simulink library "dspsigattribs"  (Simulink 8.0)
settings: Solver=ode45  SolverMode=SingleTasking  StartTime=0.0  StopTime=10.0  RelTol=1e-3
values from neighbouring files (symbols this model uses):
  D = D + B    [rebuffer_delay.m]
libraries: simulink x2
settings Model: RequirementInfo=9  Creator=don  LastModifiedBy=lij  CovMetricSettings=d  ExtModeAutoUpdateStatusClock=off
settings Model: ForwardingTableString=|
  | ||__slOldName__||dspsigattribs/Contiguous
  | Copy||__slNewName__||dspobslib/Contiguous
  | Copy||__slOldName__||dspsigattribs/Frame Status
  | Conversion||__slNewName__||dspobslib/Frame Status
  | Conversion

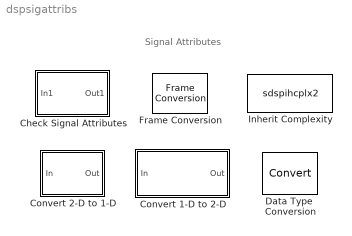
== system dspsigattribs ==
  note: Signal Attributes
  Check Signal Attributes : Subsystem  mask(Check Signal Attributes){SigAttribCheckMethod=Does not match attributes exactly, Complexity=Ignore, Frame=Ignore, DimsCheckMethod=Ignore, Dimensions=1-D, DatatypeCheckMethod=Ignore, DatatypeGeneral=Boolean, DtypeFloatSpecific=Any floating-point, DtypeFixedSpecific=Any fixed-point, DtypeIntSpecific=Any integer, SampleMode=Ignore}
      mask prompts: SigAttribCheckMethod "Error when input:"; Frame "Frame status:"; DimsCheckMethod "Dimensionality:"; DatatypeCheckMethod "Data type:"; DatatypeGeneral "General data type:"; DtypeFloatSpecific "Specific floating-point:"; DtypeFixedSpecific "Specific fixed-point:"; DtypeIntSpecific "Specific integer:"; SampleMode "Sample time:"
      mask help: Generate an error when the input signal does or does not match selected attributes exactly.
      mask Help: eval('blocksethelp');
      mask StyleString: popup(Does not match attributes exactly|Matches attributes exactly),popup(Ignore|Real|Complex),popup(Ignore|Frame-based|Sample-based),popup(Ignore|Is...|Is not...),popup(1-D|2-D|Scalar (1-D or 2-D)|Vector (1-D or 2-D)|Vector (1-D or 2-D) or scalar|Row vector (2-D)|Row vector (2-D) or scalar|Column vector (2-D)|Column vector (2-D) or scalar|Full matrix (2-D)|Square matrix (2-D)),popup(Ignore|Is...|Is not...),popup(Boolean|Enumerated|Floating-point|Floating-point or boolean|Fixed-point|Integer),popup(Any floating-point|Double precision|Single precision),popup(Any fixed-point|Signed fixed-point|Unsigned fixed-point),popup(Any integer|Signed integer|Unsigned integer|int8|int16|int32|uint8|uint16|uint32),popup(Ignore|Discrete|Continuous)
      mask CallbackString: |||dspblkchksigattrbs||dspblkchksigattrbs|dspblkchksigattrbs|||dspblkchksigattrbs|
      mask Display: disp('Check Signal\n Attributes');
  Convert 1-D to 2-D : Subsystem  mask(Convert 1-D to 2-D){M=1, N=1, frameBasedOut=off}
      mask prompts: M "Number of output rows:"; N "Number of output columns:"; frameBasedOut "Frame-based output"
      mask help: Output a (2-D) matrix signal.
      mask init:
      | dspblkcnvrt1d2d;
      mask Help: eval('blocksethelp');
      mask Display: disp('reshape(U,M,N)')
  Convert 2-D to 1-D : Subsystem
      mask Type: Convert 2-D to 1-D
      mask Description: Output a (1-D) vector signal.
      mask Help: eval('blocksethelp');
      mask Display: disp('U( : )')
  Data Type  Conversion : DataTypeConversion
  Frame Conversion : FrameConversion
  Inherit Complexity : S-Function  FunctionName=sdspihcplx2  EnableBusSupport=off
      mask Type: Inherit Complexity
      mask Description: Copy data from the Data input with the complexity of the reference signal. If the data is real and the reference is complex, an all zero imaginary part is created. If the data is complex and the reference is real, the imaginary part of the input is removed.
      mask Help: eval('blocksethelp');
      mask Display:
      | text(.9,0.5,'Inherit\nComplexity','horiz','right');
      | port_label('input',1,'Data');
      | port_label('input',2,'Ref');

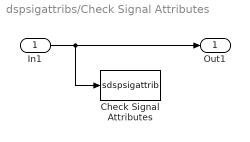
== system dspsigattribs/Check Signal Attributes ==
  In1 : Inport
  Check Signal Attributes : S-Function  FunctionName=sdspsigattrib  Parameters=SigAttribCheckMethod,Complexity,Frame,DimsCheckMethod,Dimensions,DatatypeCheckMethod,DatatypeGeneral,DtypeFloatSpecific,DtypeFixedSpecific,DtypeIntSpecific,SampleMode  EnableBusSupport=off
      mask Type: Check Signal Attributes
  Out1 : Outport
  wires:
  In1/1 -> Out1/1, Check Signal Attributes/1

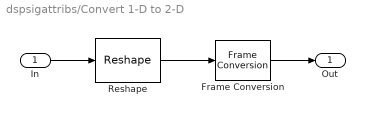
== system dspsigattribs/Convert 1-D to 2-D ==
  In : Inport
  Frame Conversion : FrameConversion  OutFrame=Sample-based
  Reshape : simulink/Math Operations/Reshape  OutputDimensionality=Customize  OutputDimensions=[M,N]
  Out : Outport
  wires:
  Frame Conversion/1 -> Out/1
  In/1 -> Reshape/1
  Reshape/1 -> Frame Conversion/1

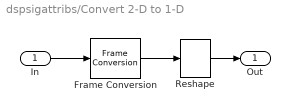
== system dspsigattribs/Convert 2-D to 1-D ==
  In : Inport
  Frame Conversion : FrameConversion  OutFrame=Sample-based
  Reshape : simulink/Math Operations/Reshape  OutputDimensionality=1-D array  OutputDimensions=[1,1]
  Out : Outport
  wires:
  Reshape/1 -> Out/1
  In/1 -> Frame Conversion/1
  Frame Conversion/1 -> Reshape/1
